simulink model "mainModel_matlab2013b_working_attitude_Tetrahedral"  (R2017a)
settings: Solver=VariableStepAuto  StartTime=0.0  StopTime=1000  MaxStep=0.01  RelTol=1e-6
settings Model: SimulationMode=rapid-accelerator  Creator=manoj  LastModifiedBy=manoj
settings DataIOCC: SaveFormat=StructureWithTime
settings OptimizationCC: LifeSpan=inf
settings DebuggingCC: AllowSymbolicDim=off  SFExecutionAtInitializationDiag=none
settings HardwareCC: ProdBitPerSizeT=32  ProdBitPerPtrDiffT=32  ProdWordSize=32  ProdHWDeviceType=Specified

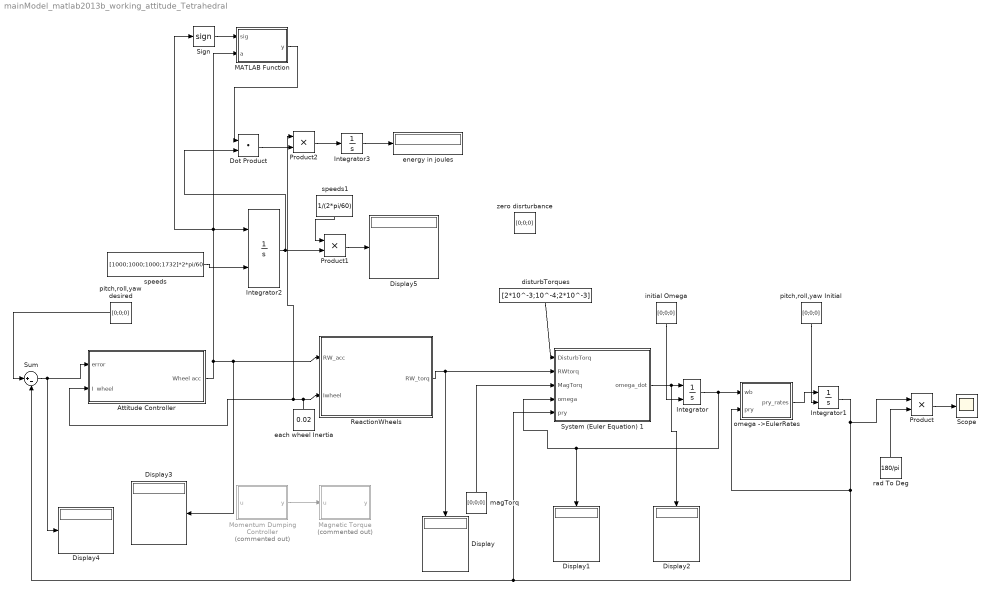
== system mainModel_matlab2013b_working_attitude_Tetrahedral ==
  Attitude Controller : Subsystem
  Display{,1..5} (6 alike) : Display
  Dot Product : DotProduct  InputSameDT=on  OutDataTypeStr=Inherit: Inherit via internal rule
  Integrator : Integrator  InitialConditionSource=external
  Integrator1 : Integrator  InitialConditionSource=external
  Integrator2 : Integrator  InitialConditionSource=external  LimitOutput=on  UpperSaturationLimit=3000*2*pi/60  LowerSaturationLimit=50*2*pi/60  ShowStatePort=on
  Integrator3 : Integrator
  MATLAB Function : MATLAB Function  TreatAsAtomicUnit=on
  "Magnetic Torque " : MATLAB Function  Commented=on  TreatAsAtomicUnit=on
  Momentum Dumping Controller : MATLAB Function  Commented=on  TreatAsAtomicUnit=on
  Product : Product
  Product1 : Product
  Product2 : Product
  ReactionWheels : MATLAB Function  TreatAsAtomicUnit=on
  Scope : Scope
  Sign : Signum
  Sum : Sum  Inputs=|+-
  System (Euler Equation) 1 : MATLAB Function  TreatAsAtomicUnit=on
  disturbTorques : Constant  Value=[2*10^-3;10^-4;2*10^-3]
  each wheel Inertia : Constant  Value=0.02
  energy in joules : Display
  initial Omega : Constant  Value=[0;0;0]
  "magTorq " : Constant  Value=[0;0;0]
  omega ->EulerRates : MATLAB Function  TreatAsAtomicUnit=on
  pitch,roll,yaw Initial : Constant  Value=[0;0;0]
  pitch,roll,yaw desired : Constant  Value=[0;0;0]
  rad To Deg : Constant  Value=180/pi
  speeds : Constant  Value=[1000;1000;1000;1732]*2*pi/60
  speeds1 : Constant  Value=1/(2*pi/60)
  "zero disrturbance " : Constant  Value=[0;0;0]
  wires:
  Momentum Dumping Controller/1(y) -> "Magnetic Torque "/1(u)
  each wheel Inertia/1 -> Product2/1, Attitude Controller/2(I  wheel), ReactionWheels/2(Iwheel)
  speeds/1 -> Integrator2/2
  Integrator/1 -> System (Euler Equation) 1/4(omega), Display1/1, omega ->EulerRates/1(wb)
  Integrator1/1 -> Product/1, omega ->EulerRates/2(pry), System (Euler Equation) 1/5(pry), Sum/2
  ReactionWheels/1(RW_torq) -> System (Euler Equation) 1/2(RWtorq), Display/1
  omega ->EulerRates/1(pry_rates) -> Integrator1/1
  "magTorq "/1 -> System (Euler Equation) 1/3(MagTorq)
  initial Omega/1 -> Integrator/2
  pitch,roll,yaw Initial/1 -> Integrator1/2
  Product/1 -> Scope/1
  rad To Deg/1 -> Product/2
  System (Euler Equation) 1/1(omega_dot) -> Display2/1, Integrator/1
  pitch,roll,yaw desired/1 -> Sum/1
  Sum/1 -> Display4/1, Attitude Controller/1(error)
  disturbTorques/1 -> System (Euler Equation) 1/1(DisturbTorq)
  Product1/1 -> Display5/1
  Integrator2/1 -> Product1/2, Dot Product/2
  speeds1/1 -> Product1/1
  Dot Product/1 -> Product2/2
  Product2/1 -> Integrator3/1
  Integrator3/1 -> energy in joules/1
  MATLAB Function/1(y) -> Dot Product/1
  Sign/1 -> MATLAB Function/1(sig)
  Attitude Controller/1(Wheel acc) -> MATLAB Function/2(a), Sign/1, Integrator2/1, ReactionWheels/1(RW_acc), Display3/1

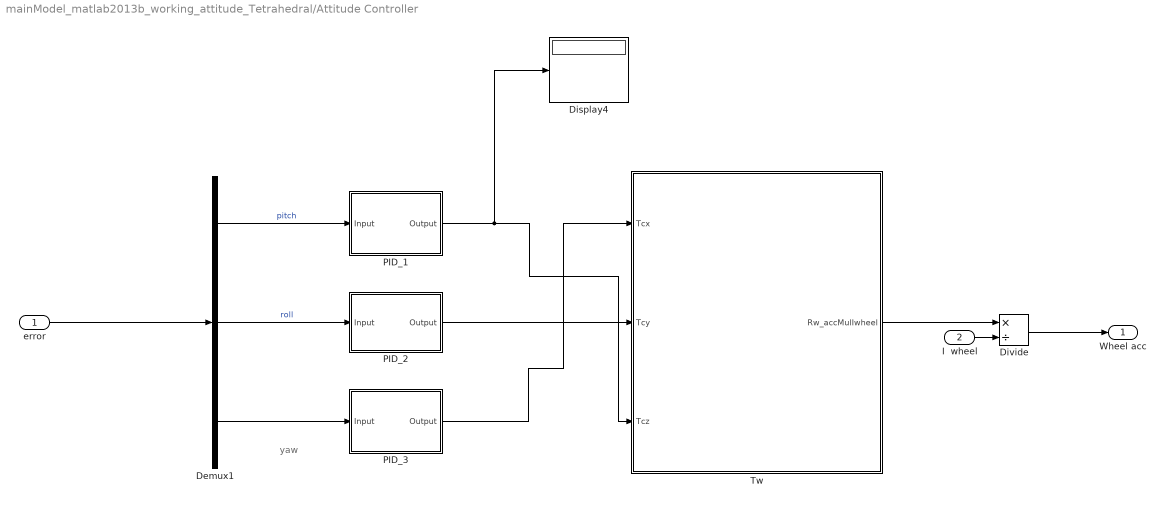
== system mainModel_matlab2013b_working_attitude_Tetrahedral/Attitude Controller ==
  note: yaw
  error : Inport
  I  wheel : Inport  Port=2
  Demux1 : Demux  Outputs=3
  Display4 : Display
  Divide : Product  Inputs=*/
  PID_1 : Subsystem
  PID_2 : Subsystem
  PID_3 : Subsystem
  "Tw " : MATLAB Function  TreatAsAtomicUnit=on
  Wheel acc : Outport
  wires:
  error/1 -> Demux1/1
  Demux1/1 -> PID_1/1(Input)  "pitch"
  PID_1/1(Output) -> "Tw "/3(Tcz), Display4/1
  Demux1/2 -> PID_2/1(Input)  "roll"
  PID_2/1(Output) -> "Tw "/2(Tcy)
  Demux1/3 -> PID_3/1(Input)
  I  wheel/1 -> Divide/2
  Divide/1 -> Wheel acc/1
  "Tw "/1(Rw_accMulIwheel) -> Divide/1
  PID_3/1(Output) -> "Tw "/1(Tcx)

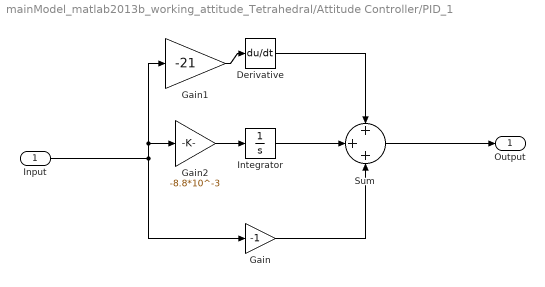
== system mainModel_matlab2013b_working_attitude_Tetrahedral/Attitude Controller/PID_1 ==
  Input : Inport
  Derivative : Derivative  CoefficientInTFapproximation=0
  Gain : Gain  Gain=-1
  Gain1 : Gain  Gain=-21
  Gain2 : Gain  Gain=-8.8*10^-3
  Integrator : Integrator
  Sum : Sum  Inputs=+++
  Output : Outport
  wires:
  Gain1/1 -> Derivative/1
  Integrator/1 -> Sum/2
  Sum/1 -> Output/1
  Gain2/1 -> Integrator/1
  Derivative/1 -> Sum/1
  Gain/1 -> Sum/3
  Input/1 -> Gain1/1, Gain2/1, Gain/1

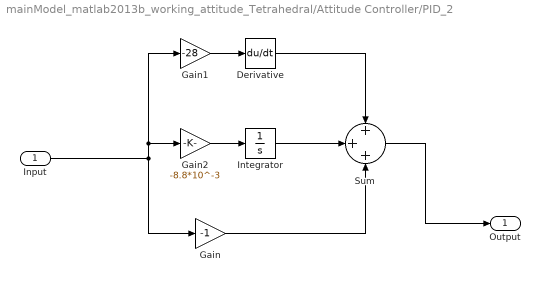
== system mainModel_matlab2013b_working_attitude_Tetrahedral/Attitude Controller/PID_2 ==
  Input : Inport
  Derivative : Derivative  CoefficientInTFapproximation=0
  Gain : Gain  Gain=-1
  Gain1 : Gain  Gain=-28
  Gain2 : Gain  Gain=-8.8*10^-3
  Integrator : Integrator
  Sum : Sum  Inputs=+++
  Output : Outport
  wires:
  Gain1/1 -> Derivative/1
  Integrator/1 -> Sum/2
  Sum/1 -> Output/1
  Gain2/1 -> Integrator/1
  Derivative/1 -> Sum/1
  Gain/1 -> Sum/3
  Input/1 -> Gain1/1, Gain2/1, Gain/1

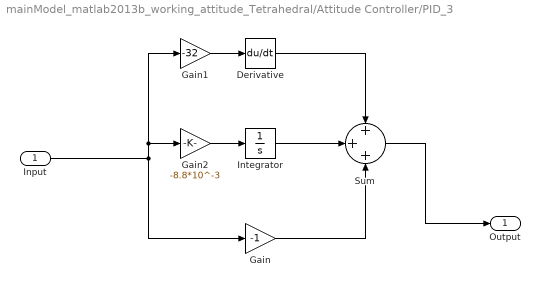
== system mainModel_matlab2013b_working_attitude_Tetrahedral/Attitude Controller/PID_3 ==
  Input : Inport
  Derivative : Derivative  CoefficientInTFapproximation=0
  Gain : Gain  Gain=-1
  Gain1 : Gain  Gain=-32
  Gain2 : Gain  Gain=-8.8*10^-3
  Integrator : Integrator
  Sum : Sum  Inputs=+++
  Output : Outport
  wires:
  Gain1/1 -> Derivative/1
  Integrator/1 -> Sum/2
  Sum/1 -> Output/1
  Gain2/1 -> Integrator/1
  Derivative/1 -> Sum/1
  Gain/1 -> Sum/3
  Input/1 -> Gain1/1, Gain2/1, Gain/1

== matlab function mainModel_matlab2013b_working_attitude_Tetrahedral/Attitude Controller/Tw  ==
  data: Tcx input; Tcy input; Rw_accMulIwheel output; Tcz input
function Rw_accMulIwheel = fcn(Tcx,Tcy,Tcz)
%Rw_acc=[0;0;0;0]; %no controller for now. This acceleration correspond
% to the rate of change in speed of each wheel. wheel speeds are always
% positive buy convention
Tc = [Tcx;Tcy;Tcz];

Conv=0.25*[sqrt(3),sqrt(3),sqrt(3)
           -sqrt(3),-sqrt(3),sqrt(3)
           -sqrt(3),sqrt(3),-sqrt(3)
           sqrt(3),-sqrt(3),-sqrt(3)];

Rw_accMulIwheel = Conv*Tc;
end

== matlab function mainModel_matlab2013b_working_attitude_Tetrahedral/MATLAB Function ==
  data: sig input; y output; a input
function y = fcn(sig,a)
y=sig.*a;
end

== matlab function mainModel_matlab2013b_working_attitude_Tetrahedral/System (Euler Equation) 1 ==
  data: DisturbTorq input; RWtorq input; omega_dot output; MagTorq input; omega input; pry input
function omega_dot = fcn( DisturbTorq,RWtorq,MagTorq,omega,pry)
%[x,y,z] corresponds to yaw roll and pitch axis!!!
%omega written here is wrt orbit and written in body frame
MOI=[1800 -50 -15;-50 1600 25;-15 25 1200];%momentOfInertia of Satellite(with everything)
%Mass=1600;%kg
p=pry(1);
r=pry(2);
y=pry(3);
Cx=[    1, 0, 0
        0, cos(y), sin(y)
        0, -sin(y), cos(y)];

Cy=[    cos(r), 0, -sin(r);
        0, 1, 0;
        sin(r), 0, cos(r) ];

Cz=[    cos(p), sin(p), 0;
        -sin(p), cos(p), 0;
        0, 0, 1    ];
Cbo=Cx*Cy*Cz; %orbit to body frame matrix adopting 3,2,1 convention on (x,y,z)
Wo=1.0741*10^-3;
temp1=(omega-Cbo*[0;0;Wo]);
temp2=cross(omega,Cbo*[0;0;Wo]);
omega_dot=(MOI)\(DisturbTorq+MagTorq-RWtorq-cross(temp1,MOI*temp1))-temp2;

end

== matlab function mainModel_matlab2013b_working_attitude_Tetrahedral/Magnetic Torque  ==
  data: u input; y output
function y = fcn(u)

y = u;

== matlab function mainModel_matlab2013b_working_attitude_Tetrahedral/omega ->EulerRates ==
  data: wb input; pry_rates output; pry input
function pry_rates  = fcn(wb,pry)
%[x,y,z] 3-2-1 rotation, where x=yaw,y=roll,z=pitch axis
% pry-pitch,yaw,roll angles

% Cx=[    1, 0, 0
%         0, cos(yaw), sin(yaw)
%         0, -sin(yaw), cos(yaw)    ];
% 
% Cy=[    cos(roll), 0, -sin(roll);
%         0, 1, 0;
%         sin(roll), 0, cos(roll) ];
% 
% Cz=[    cos(pitch), sin(pitch), 0;
%         -sin(pitch), cos(pitch), 0;
%         0, 0, 1    ];NOT NEEDED HERE BUT CAN BE USED ELSEWHERE IF NEEDEd

%p=pry(1);
r=pry(2);
y=pry(3);
C_pryToOmega=   [   -sin(r),        0,      1
                    cos(r)*sin(y),  cos(y), 0
                    cos(r)*cos(y), -sin(y), 0];
pry_rates=(C_pryToOmega)\wb;

== matlab function mainModel_matlab2013b_working_attitude_Tetrahedral/ReactionWheels ==
  data: RW_acc input; RW_torq output size=3; Iwheel input
function RW_torq = fcn(RW_acc,Iwheel)
%For the tetrahedron one
%RW_acc means acceleration of 4 individual wheel speeds

RW_torq=Iwheel*[1/sqrt(3),-1/sqrt(3),-1/sqrt(3),1/sqrt(3)
                1/sqrt(3),-1/sqrt(3),1/sqrt(3),-1/sqrt(3)
                1/sqrt(3),1/sqrt(3),-1/sqrt(3),-1/sqrt(3)]*RW_acc;
% if speedLimitSituation~=0
%     RW_torq=Torq_acceleration_part;       
% else
%     RW_torq=[0;0;0]; %considering saturation of wheels into account
end

== matlab function mainModel_matlab2013b_working_attitude_Tetrahedral/Momentum Dumping Controller ==
  data: u input; y output
function y = fcn(u)

y = u;
